simulink model "SimModel"  (R2020b)
settings: Solver=VariableStepAuto  StartTime=0.0  StopTime=10.0  MaxStep=0.01  RelTol=1e-3
libraries: fuzblock x1
settings Model: Creator=Armin  LastModifiedBy=Armin

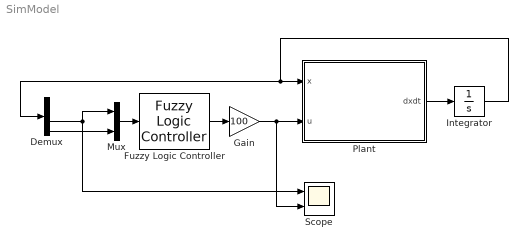
== system SimModel ==
  Demux : Demux
  Fuzzy Logic Controller : fuzblock/Fuzzy Logic  Controller  FIS='InvPendulum.fis'  OutputSampleNumber=101  DataType=double  FuzzifiedInputs=off  RuleFiringStrengths=off  RuleOutputs=off  AggregatedOutputs=off  SimulateUsing=Interpreted execution  OutOfRangeInputValueMessage=warning  NoRuleFiredMessage=warning  EmptyOutputFuzzySetMessage=warning
  Gain : Gain  Gain=100
  Integrator : Integrator  InitialCondition=[0 0 0.2 0]
  Mux : Mux  Inputs=2
  Plant : MATLAB Function  TreatAsAtomicUnit=on
  Scope : Scope  NumInputPorts=2
  wires:
  Plant/1(dxdt) -> Integrator/1
  Integrator/1 -> Demux/1, Plant/1(x)
  Mux/1 -> Fuzzy Logic Controller/1
  Demux/3 -> Mux/1, Scope/1
  Demux/4 -> Mux/2
  Fuzzy Logic Controller/1 -> Gain/1
  Gain/1 -> Scope/2, Plant/2(u)

== matlab function SimModel/Plant ==
  data: x input; u input; dxdt output
function dxdt = Model(x,u)
dxdt = zeros(4,1);

x1 = x(1);
x2 = x(2);
x3 = x(3);
x4 = x(4);

M = 2;
m = 1;
l = 1;
g = 9.81;
ft = 0.5;

dxdt(1) = x2;
dxdt(2) = (-m*g*sin(x3)*cos(x3) + m*l*x4^2*sin(x3) + ft*m*x4*cos(x3) + u)/(M + (1 - cos(x3)^2)*m);
dxdt(3) = x4;
dxdt(4) = ((M + m)*(g*sin(x3) - ft*x4) - (l*m*x4^2*sin(x3) + u)*cos(x3))/(l*(M + (1 - cos(x3)^2)*m));
end
